simulink model "Thesis_VehicleModel_MPC_ECMS"  (R2018b)
settings: Solver=FixedStepAuto  StartTime=0.0  StopTime=10  FixedStep=0.01  RelTol=1e-5
PostLoadFcn:
  | , if any(exist('dsrtsu_mdlpostloadfcn', 'file') == [2, 3, 6]), try dsrtsu_mdlpostloadfcn('Execute', bdroot); catch fprintf('Error in PostLoadFcn (dsrtsu_mdlpostloadfcn) for model "%s":\n %s\n', bdroot, lasterr); end, end,
InitFcn:
  | clc;clear all;
model workspace (MAT data in the model file):
  MDL : struct (value not decoded)
values from neighbouring files (symbols this model uses):
  MDL =     [MDL.mat]
libraries: simulink x14, rtican x9, autolibshared x1, mpclib x1
(part 2 of 5)

== system Thesis_VehicleModel_MPC_ECMS/Genset Powertrain Dynamics2/Generator ==
  MechPwrIn(W) : Inport
  GensetCmd : Inport  Port=2
  Power Setpoint : Inport  Port=3
  Constant1 : Constant  Value=0
  Constant2 : Constant  Value=0
  Current Servo System : TransferFcn  Denominator=[0.2 1]
  Load Torque Servo System : TransferFcn  Denominator=[0.2 1]
  Product : Product
  Saturation : Saturate  UpperLimit=70  LowerLimit=0
  Saturation Dynamic : simulink/Discontinuities/Saturation Dynamic  OutMin=[]  OutMax=[]  OutDataTypeStr=Inherit: Same as second input  OutDataType=fixdt(1, 16)  OutScaling=2^-10  DoSatur=off
  Saturation Dynamic1 : simulink/Discontinuities/Saturation Dynamic  OutMin=[]  OutMax=[]  OutDataTypeStr=Inherit: Same as second input  OutDataType=fixdt(1, 16)  OutScaling=2^-10  DoSatur=off
  Saturation1 : Saturate  UpperLimit=inf  LowerLimit=0
  Subsystem : Subsystem
  Subtract : Sum  Inputs=+-
  Terminator : Terminator
  Thermal Contraint : Subsystem
  "Voltage, Current and Load Torque Mapping" : MATLAB Function  TreatAsAtomicUnit=on
  GenPwrOut (W) : Outport
  "Torque_Load " : Outport  Port=2
  MaxMechPwr : Outport  Port=3
  wires:
  GensetCmd/1 -> Subsystem/2("Genset Cmd ")
  Constant1/1 -> Saturation Dynamic/3
  Saturation Dynamic1/1 -> GenPwrOut (W)/1  "GenPwrOut (W)"
  Saturation Dynamic/1 -> Subtract/1, Subsystem/1(Mech_Pwr), Thermal Contraint/1(MechPwrIn)
  Thermal Contraint/1(MaxMechPwr) -> MaxMechPwr/1, Saturation Dynamic/1
  MechPwrIn(W)/1 -> Saturation Dynamic/2
  Subsystem/1(Pwr_Loss) -> Subtract/2  "Gen Pwr Loss"
  "Voltage, Current and Load Torque Mapping"/3(LoadTorque) -> Saturation/1  "T_load*"
  Load Torque Servo System/1 -> "Torque_Load "/1  "T_load"
  "Voltage, Current and Load Torque Mapping"/2(Current) -> Current Servo System/1  "Current*"
  Power Setpoint/1 -> "Voltage, Current and Load Torque Mapping"/1(P)  "Power_cmd"
  Saturation/1 -> Load Torque Servo System/1
  Constant2/1 -> Saturation Dynamic1/3
  Product/1 -> Saturation Dynamic1/2
  "Voltage, Current and Load Torque Mapping"/1(Volt) -> Product/2
  Current Servo System/1 -> Terminator/1, Product/1  "Current"
  Subtract/1 -> Saturation1/1
  Saturation1/1 -> Saturation Dynamic1/1  "Gen Upper Bound"

== system Thesis_VehicleModel_MPC_ECMS/Genset Powertrain Dynamics2/Power//rpm Setpoints ==
  Power Command : Inport
  Genset Cmd : Inport  Port=2
  Chart : Stateflow chart  TreatAsAtomicUnit=on
  Clock : Clock
  MATLAB Function : MATLAB Function  TreatAsAtomicUnit=on
  Power Setpoint : Outport
  rpm Setpoint : Outport  Port=2
  wires:
  Power Command/1 -> MATLAB Function/1(Power_Cmd)
  Clock/1 -> Chart/2(t)
  MATLAB Function/1(PowerSetPoint) -> Chart/1(PowerSetPoint)
  MATLAB Function/2(rpmSetPoint) -> Chart/3(rpmSetPoint)
  Chart/2(PowerCmd) -> Power Setpoint/1
  Chart/1(rpmCmd) -> rpm Setpoint/1
  Genset Cmd/1 -> MATLAB Function/2(GensetCmd)

== system Thesis_VehicleModel_MPC_ECMS/Genset Powertrain Dynamics2/Rpm Controller ==
  Engine rpm : Inport
  rpm setpoint : Inport  Port=2
  Engine Power Set Point : Inport  Port=3
  Calculate Feedback Mapping : Product  Multiplication=Matrix(*)
  Calculate Fix Point : Subsystem
  Demux : Demux  Outputs=2
  Gain : Gain  Gain=30/pi
  Kalman Filter : Subsystem
  LQG Gain Mapping : MATLAB Function  TreatAsAtomicUnit=on
  Noise : RandomNumber  Variance=300  SampleTime=0.1
  Scope : Scope
  Scope1 : Scope
  Sum : Sum  Inputs=|-+
  Sum1 : Sum  Inputs=|++
  Sum2 : Sum  Inputs=|++
  TPS limit : Saturate  UpperLimit=0.98  LowerLimit=0
  Terminator : Terminator
  dSPACE CANBUS Protocol : Subsystem  Commented=on
  rpm regulation : Stateflow chart  Commented=on  TreatAsAtomicUnit=on
  rpm2rads1 : Gain  Gain=pi/30
  TPS Command : Outport
  wires:
  Sum2/1 -> LQG Gain Mapping/1(rpm), rpm2rads1/1, Kalman Filter/2("rpm ")  "Engine rpm with noise"
  Kalman Filter/1("x_hat ") -> Scope/1, Sum/2, Gain/1  "State Estimation x_hat"
  Sum/1 -> Calculate Feedback Mapping/2
  Sum1/1 -> Kalman Filter/3(u)
  rpm2rads1/1 -> Kalman Filter/1(y)
  TPS limit/1 -> Sum1/2, TPS Command/1
  LQG Gain Mapping/2(gain) -> Calculate Feedback Mapping/1
  Engine rpm/1 -> Sum2/1
  Noise/1 -> Sum2/2
  LQG Gain Mapping/1(comp) -> Sum1/1
  rpm setpoint/1 -> Calculate Fix Point/1(rpm set point)
  Calculate Fix Point/1(rpm_cmd) -> LQG Gain Mapping/2(rpm_cmd)
  Calculate Fix Point/2(fix point (2 states)) -> Sum/1
  Engine Power Set Point/1 -> LQG Gain Mapping/3(PowerSetPoint)
  Calculate Feedback Mapping/1 -> TPS limit/1
  Gain/1 -> Demux/1
  Demux/1 -> Scope1/1
  Demux/2 -> Terminator/1

== system Thesis_VehicleModel_MPC_ECMS/RTI Data/RTI Data Store ==
  RTI Data Store : Subsystem  mask(RTI_DATA_STORE){}
      mask help:
      | RTI Data Store Block. This block is used by RTI to store internal model dependent data. Deleting this block will result in data loss.
      |
      | NEVER DELETE, COPY, OR MODIFY THIS BLOCK!
      mask Help:
      | RTI Data Store Block. This block is used by RTI to store internal model dependent data. Deleting this block will result in data loss.
      | 
      | NEVER DELETE, COPY, OR MODIFY THIS BLOCK!
      mask Display: text(0.5, 0.5, ' ', 'HorizontalAlignment', 'center');

== system Thesis_VehicleModel_MPC_ECMS/Supervisory Control MPC Archive/Nonlinear_MPC ==
  SOC : Inport
  SOC_ref : Inport  Port=2
  Measured Disturbance : Inport  Port=3
  Nonlinear MPC Controller1 : mpclib/Nonlinear MPC Controller  SCDEnableBlockLinearizationSpecification=on  nlmpcobj=Pw_Trobj  UseObjectTs=on  md_enabled=on  param_enabled=off  cost_enabled=on  mvseq_enabled=off  stateseq_enabled=off  ovseq_enabled=off  slack_enabled=off  status_enabled=on  ov_min=off  ov_max=off  mv_min=off  mv_max=off  mvrate_min=off  mvrate_max=off  state_min=off  state_max=off  ov_weight=off  mv_weight=off  mvrate_weight=off  ecr_weight=off  mvtarget_enabled=off  nlp_initialize=off
      settings: SourceProductName=Model Predictive Control Toolbox
  Terminator : Terminator
  Terminator1 : Terminator
  Unit Delay1 : UnitDelay  SampleTime=-1
  Manipulated Variable : Outport
  wires:
  Nonlinear MPC Controller1/1 -> Manipulated Variable/1, Unit Delay1/1
  Unit Delay1/1 -> Nonlinear MPC Controller1/3
  SOC/1 -> Nonlinear MPC Controller1/1
  SOC_ref/1 -> Nonlinear MPC Controller1/2
  Measured Disturbance/1 -> Nonlinear MPC Controller1/4
  Nonlinear MPC Controller1/2 -> Terminator/1  "MPC Optimal Cost"
  Nonlinear MPC Controller1/3 -> Terminator1/1  "MPC Status"

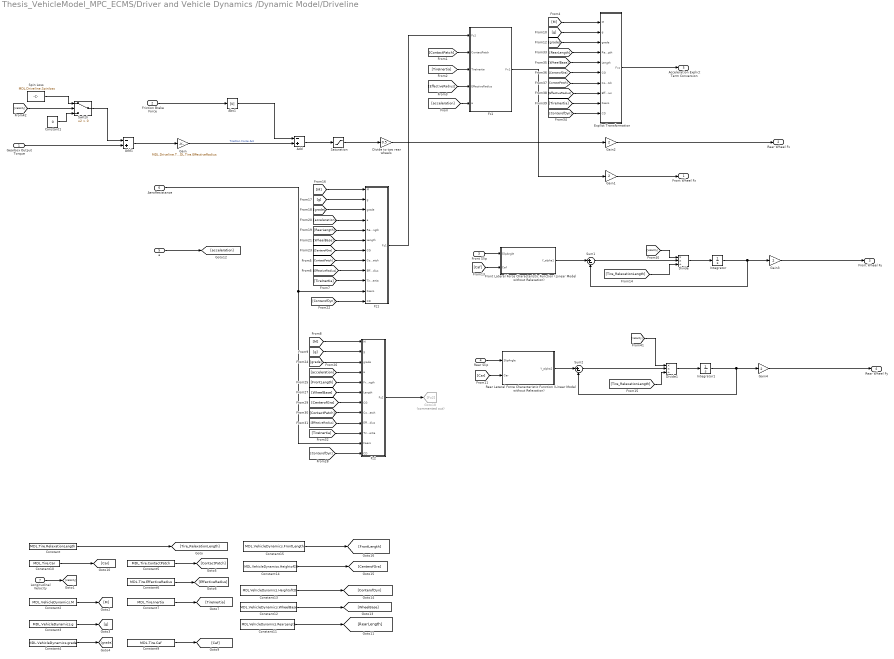
== system Thesis_VehicleModel_MPC_ECMS/Driver and Vehicle Dynamics /Dynamic Model/Driveline ==
  Gearbox Output Torque : Inport
  Friction Brake Force : Inport  Port=2
  Front Slip : Inport  Port=3
  Rear Slip : Inport  Port=4
  a : Inport  Port=5
  "AeroResistance " : Inport  Port=6
  Longitudinal Velocity : Inport  Port=7
  Abs1 : Abs
  Add : Sum  Inputs=-+
  Add1 : Sum  Inputs=-+
  Constant : Constant  Value=MDL.Tire.RelaxationLength
  Constant1 : Constant  Value=0
  Constant10 : Constant  Value=MDL.Tire.Car
  Constant11 : Constant  Value=MDL.VehicleDynamics.RearLength
  Constant12 : Constant  Value=MDL.VehicleDynamics.WheelBase
  Constant13 : Constant  Value=MDL.VehicleDynamics.HeightofCD
  Constant14 : Constant  Value=MDL.VehicleDynamics.HeightofCG
  Constant15 : Constant  Value=MDL.VehicleDynamics.FrontLength
  Constant2 : Constant  Value=MDL.VehicleDynamics.M
  Constant3 : Constant  Value=MDL.VehicleDynamics.g
  Constant4 : Constant  Value=MDL.VehicleDynamics.grade
  Constant5 : Constant  Value=MDL.Tire.ContactPatch
  Constant6 : Constant  Value=MDL.Tire.EffectiveRadius
  Constant7 : Constant  Value=MDL.Tire.Inertia
  Constant9 : Constant  Value=MDL.Tire.Caf
  Divide : Product  Inputs=**/
  Divide to two rear wheels : Gain  Gain=0.5
  Divide1 : Product  Inputs=**/
  Explict Transformation : MATLAB Function  TreatAsAtomicUnit=on
  Front Lateral Force Characteristic Function (Linear Model without Relexation) : MATLAB Function  TreatAsAtomicUnit=on
  Fx1 : MATLAB Function  TreatAsAtomicUnit=on
  Fz1 : MATLAB Function  TreatAsAtomicUnit=on
  Fz2 : MATLAB Function  TreatAsAtomicUnit=on
  Gain : Gain  Gain=MDL.Driveline.TFRatio/MDL.Tire.EffectiveRadius
  Gain{1..4} (4 alike) : Gain  Gain=2
  Goto18 : Goto  Commented=on  GotoTag=Fz2
  Integrator : Integrator
  Integrator1 : Integrator
  Rear Lateral Force Characteristic Function (Linear Model without Relexation) : MATLAB Function  TreatAsAtomicUnit=on
  Saturation : Saturate  UpperLimit=MDL.Driveline.MaxTrac  LowerLimit=-MDL.Driveline.MaxTrac
  Spin Loss : Constant  Value=MDL.Driveline.Spinloss
  Sum1 : Sum  Inputs=|+-
  Sum2 : Sum  Inputs=|+-
  Switch : Switch  Criteria=u2 > Threshold
  "Front Wheel Fx " : Outport
  Rear Wheel Fx : Outport  Port=2
  Front Wheel Fy : Outport  Port=3
  Rear Wheel Fy : Outport  Port=4
  Acceleration Explict Term Conversion : Outport  Port=5
  wires:
  Gearbox Output Torque/1 -> Add1/2
  Divide to two rear wheels/1 -> Gain2/1
  Front Slip/1 -> Front Lateral Force Characteristic Function (Linear Model without Relexation)/1(SlipAngle)
  Rear Slip/1 -> Rear Lateral Force Characteristic Function (Linear Model without Relexation)/1(SlipAngle)
  Gain1/1 -> "Front Wheel Fx "/1
  Gain2/1 -> Rear Wheel Fx/1
  Constant2/1 -> [M]
  Constant3/1 -> [g]
  Constant4/1 -> [grade]
  Constant5/1 -> [ContactPatch]
  Constant6/1 -> [EffectiveRadius]
  Constant7/1 -> [TireInertia]
  [ContactPatch] -> Fz1/8(ContactPatch)
  [EffectiveRadius] -> Fz1/9(EffectiveRadius)
  [TireInertia] -> Fz1/10(TireInertia)
  Constant9/1 -> [Caf]
  [Car] -> Rear Lateral Force Characteristic Function (Linear Model without Relexation)/2(Car)
  [Caf] -> Front Lateral Force Characteristic Function (Linear Model without Relexation)/2(Caf)
  Constant10/1 -> [Car]
  [M] -> Fz1/1(M)
  [g] -> Fz1/2(g)
  [grade] -> Fz1/3(grade)
  Constant11/1 -> [RearLength]
  [RearLength] -> Fz1/5(RearLength)
  [acceleration] -> Fz1/4(a)
  Constant12/1 -> [WheelBase]
  [WheelBase] -> Fz1/6(Length)
  Constant13/1 -> [ConterofDyn]
  [ConterofDyn] -> Fz1/12(CD)
  Constant14/1 -> [CenterofGra]
  [CenterofGra] -> Fz1/7(CG)
  [M] -> Fz2/1(M)
  [grade] -> Fz2/3(grade)
  [CenterofGra] -> Fz2/7(CG)
  [FrontLength] -> Fz2/5(FrontLength)
  [g] -> Fz2/2(g)
  [WheelBase] -> Fz2/6(Length)
  [EffectiveRadius] -> Fz2/9(EffectiveRadius)
  [ConterofDyn] -> Fz2/12(CD)
  [ContactPatch] -> Fz2/8(ContactPatch)
  [TireInertia] -> Fz2/10(TireInertia)
  [acceleration] -> Fz2/4(a)
  Constant15/1 -> [FrontLength]
  [ContactPatch] -> Fx1/2(ContactPatch)
  [TireInertia] -> Fx1/3(TireInertia)
  [EffectiveRadius] -> Fx1/4(EffectiveRadius)
  Fx1/1(Fx1) -> Gain1/1
  a/1 -> [acceleration]
  "AeroResistance "/1 -> Fz1/11(Faero), Fz2/11(Faero)
  Fz1/1(Fz1) -> Fx1/1(Fz1)
  [acceleration] -> Fx1/5(a)
  [M] -> Explict Transformation/1(M)
  [g] -> Explict Transformation/2(g)
  [grade] -> Explict Transformation/3(grade)
  [RearLength] -> Explict Transformation/4(RearLength)
  [WheelBase] -> Explict Transformation/5(Length)
  [CenterofGra] -> Explict Transformation/6(CG)
  [ContactPatch] -> Explict Transformation/7(ContactPatch)
  [EffectiveRadius] -> Explict Transformation/8(EffectiveRadius)
  [TireInertia] -> Explict Transformation/9(Faero)
  [ConterofDyn] -> Explict Transformation/10(CD)
  Explict Transformation/1(Fxs) -> Acceleration Explict Term Conversion/1
  Fz2/1(Fz2) -> Goto18/1
  Gain/1 -> Add/2  "Traction Force Acc"
  Integrator/1 -> Sum1/2, Gain3/1
  Front Lateral Force Characteristic Function (Linear Model without Relexation)/1(Y_alpha1) -> Sum1/1
  Constant/1 -> [Tire_RelexationLength]
  Sum1/1 -> Divide/2
  Divide/1 -> Integrator/1
  Gain3/1 -> Front Wheel Fy/1
  Integrator1/1 -> Sum2/2, Gain4/1
  Sum2/1 -> Divide1/2
  Divide1/1 -> Integrator1/1
  Rear Lateral Force Characteristic Function (Linear Model without Relexation)/1(Y_alpha2) -> Sum2/1
  Gain4/1 -> Rear Wheel Fy/1
  [Tire_RelexationLength] -> Divide1/3
  [Tire_RelexationLength] -> Divide/3
  [Velocity] -> Divide/1
  Longitudinal Velocity/1 -> [Velocity]
  [Velocity] -> Divide1/1
  Friction Brake Force/1 -> Abs1/1
  Abs1/1 -> Add/1
  Add/1 -> Saturation/1
  Saturation/1 -> Divide to two rear wheels/1
  Add1/1 -> Gain/1
  [Velocity] -> Switch/2
  Constant1/1 -> Switch/3
  Switch/1 -> Add1/1
  Spin Loss/1 -> Switch/1

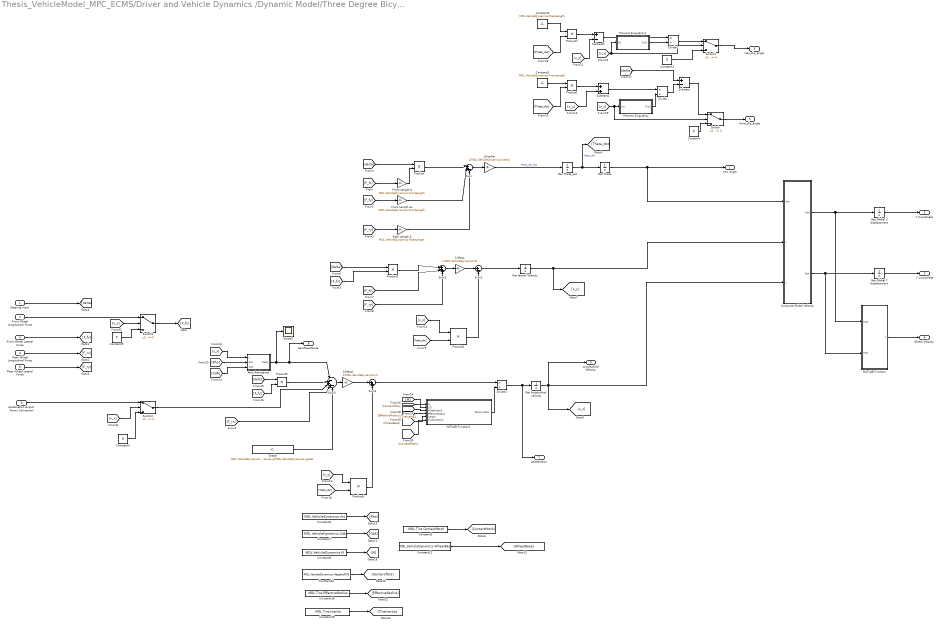
== system Thesis_VehicleModel_MPC_ECMS/Driver and Vehicle Dynamics /Dynamic Model/Three Degree Bicycle Model ==
  Steering Input : Inport
  Front Wheel Longitudinal Force : Inport  Port=2
  Rear Wheel Longitudinal Force : Inport  Port=3
  Front Wheel Lateral Force : Inport  Port=4
  Rear Wheel Lateral Force : Inport  Port=5
  Acceleration Explict Terms Conversion : Inport  Port=6
  1/Inertia : Gain  Gain=1/MDL.VehicleDynamics.Inertia
  1/Mass : Gain  Gain=1/MDL.VehicleDynamics.M
  1/Mass1 : Gain  Gain=1/MDL.VehicleDynamics.M
  Aero Resistance : MATLAB Function  TreatAsAtomicUnit=on
  Compute Global Velocity : MATLAB Function  TreatAsAtomicUnit=on
  Constant{,1,4,9} (4 alike) : Constant  Value=0
  Constant12 : Constant  Value=MDL.VehicleDynamics.WheelBase
  Constant14 : Constant  Value=MDL.VehicleDynamics.HeightofCG
  Constant18 : Constant  Value=MDL.Tire.EffectiveRadius
  Constant19 : Constant  Value=MDL.Tire.Inertia
  Constant2 : Constant  Value=MDL.VehicleDynamics.RearLength
  Constant3 : Constant  Value=MDL.VehicleDynamics.FrontLength
  Constant5 : Constant  Value=MDL.Tire.ContactPatch
  Constant6 : Constant  Value=MDL.VehicleDynamics.rho
  Constant7 : Constant  Value=MDL.VehicleDynamics.CdA
  Constant8 : Constant  Value=MDL.VehicleDynamics.M
  Divide : Product  Inputs=*/
  Divide1 : Product  Inputs=*/
  Divide2 : Product  Inputs=*/
  Front Length a : Gain  Gain=MDL.VehicleDynamics.FrontLength
  Front Length a1 : Gain  Gain=MDL.VehicleDynamics.FrontLength
  Get Global X displacement : Integrator
  Get Global Y displacement : Integrator
  Get Theta : Integrator
  Get Theta_dot : Integrator
  Get lateral Velocity : Integrator
  Get longitudinal velocity : Integrator
  Grade : Constant  Value=MDL.VehicleDynamics.M*MDL.VehicleDynamics.g*MDL.VehicleDynamics.grade
  MATLAB Function : MATLAB Function  TreatAsAtomicUnit=on
  MATLAB Function1 : MATLAB Function  TreatAsAtomicUnit=on
  Prevent Singularity : Subsystem
  Prevent Singularity1 : Subsystem
  Product{,1..3,5..7} (7 alike) : Product
  Rear Length b : Gain  Gain=MDL.VehicleDynamics.RearLength
  Scope2 : Scope
  Subtract : Sum  Inputs=+-
  Subtract1 : Sum  Inputs=+-
  Subtract2 : Sum
  Sum : Sum  Inputs=|++-
  Sum1 : Sum  Inputs=|+++
  Sum2 : Sum  Inputs=|+-
  Sum3 : Sum  Inputs=|--++-
  Sum4 : Sum  Inputs=|++
  Switch{,1..3} (4 alike) : Switch  Criteria=u2 ~= 0
  Yaw Angle : Outport
  Y Coordinate : Outport  Port=2
  X Coordinate : Outport  Port=3
  Global Velocity : Outport  Port=4
  front_slip_angle : Outport  Port=5
  rear_slip_angle : Outport  Port=6
  Acceleration : Outport  Port=7
  "AeroResistance " : Outport  Port=8
  "Longitudinal Velocity " : Outport  Port=9
  wires:
  [F_ry] -> Sum1/3
  1/Inertia/1 -> Get Theta_dot/1  "Theta_dot_dot"
  Get Theta_dot/1 -> [Theta_dot], Get Theta/1  "Theta_dot"
  Sum3/1 -> 1/Mass1/1
  [Theta_dot] -> Product3/2
  [delta] -> Product2/1
  Product2/1 -> Sum1/1
  [Theta_dot] -> Product6/2
  [v_y] -> Product6/1
  Product6/1 -> Sum4/2
  [delta] -> Product5/1
  Sum/1 -> 1/Inertia/1
  [F_fy] -> Sum1/2
  Get lateral Velocity/1 -> Compute Global Velocity/2(v), [v_y]
  Rear Wheel Longitudinal Force/1 -> [F_rx]
  [F_fy] -> Product5/2
  Steering Input/1 -> [delta]
  Front Wheel Lateral Force/1 -> [F_fy]
  [F_fx] -> Front Length a/1
  [F_fy] -> Front Length a1/1
  Front Wheel Longitudinal Force/1 -> Switch3/1
  Rear Wheel Lateral Force/1 -> [F_ry]
  Sum1/1 -> 1/Mass/1
  Get longitudinal velocity/1 -> "Longitudinal Velocity "/1, Compute Global Velocity/3(u), [v_x]
  [F_ry] -> Rear Length b/1
  Product3/1 -> Sum2/2
  [v_x] -> Product3/1
  Rear Length b/1 -> Sum/3
  1/Mass/1 -> Sum2/1
  Product/1 -> Sum/1
  Front Length a1/1 -> Sum/2
  Front Length a/1 -> Product/2
  Sum2/1 -> Get lateral Velocity/1
  Constant3/1 -> Product1/1
  [Theta_dot] -> Product1/2
  Product1/1 -> Subtract2/1
  [v_y] -> Subtract2/2
  Subtract2/1 -> Divide/1
  [v_x] -> Switch/2, Prevent Singularity/1(In1)
  [delta] -> Subtract/1
  Divide/1 -> Subtract/2
  Constant2/1 -> Product7/1
  [Theta_dot] -> Product7/2
  Product7/1 -> Subtract1/1
  [v_y] -> Subtract1/2
  Subtract1/1 -> Divide1/1
  Switch/1 -> front_slip_angle/1
  Subtract/1 -> Switch/1
  Constant/1 -> Switch/3
  Switch1/1 -> rear_slip_angle/1
  Divide1/1 -> Switch1/1
  Constant1/1 -> Switch1/3
  [delta] -> Product/1
  Get Global Y displacement/1 -> Y Coordinate/1
  Get Theta/1 -> Yaw Angle/1, Compute Global Velocity/1(Yaw)
  Compute Global Velocity/2(Ydot) -> MATLAB Function/2(Ydot), Get Global Y displacement/1
  Compute Global Velocity/1(Xdot) -> MATLAB Function/1(Xdot), Get Global X displacement/1
  Get Global X displacement/1 -> X Coordinate/1
  MATLAB Function/1(V) -> Global Velocity/1
  [v_x] -> Aero Resistance/1(u)
  [F_rx] -> Sum3/4
  Product5/1 -> Sum3/2
  Aero Resistance/1(Faero) -> Scope2/1, "AeroResistance "/1, Sum3/1
  [CdA] -> Aero Resistance/3(CdA)
  [Rho] -> Aero Resistance/2(Rho)
  1/Mass1/1 -> Sum4/1
  Constant14/1 -> [CenterofGra]
  Constant7/1 -> [CdA]
  Constant18/1 -> [EffectiveRadius]
  Constant19/1 -> [TireInertia]
  Constant8/1 -> [M]
  Constant6/1 -> [Rho]
  Divide2/1 -> Get longitudinal velocity/1, Acceleration/1
  [M] -> MATLAB Function1/1(M)
  [CenterofGra] -> MATLAB Function1/2(CG)
  [TireInertia] -> MATLAB Function1/3(WheelInertia)
  [EffectiveRadius] -> MATLAB Function1/4(EffectiveRadius)
  [WheelBase] -> MATLAB Function1/5(Length)
  Constant12/1 -> [WheelBase]
  Sum4/1 -> Divide2/1
  MATLAB Function1/1(Denominator) -> Divide2/2
  Constant5/1 -> [ContactPatch]
  [ContactPatch] -> MATLAB Function1/6(ContactPatch)
  [v_x] -> Switch1/2, Prevent Singularity1/1(In1)
  Prevent Singularity1/1(Out1) -> Divide1/2
  [v_x] -> Switch2/2
  Constant4/1 -> Switch2/3
  Switch2/1 -> Sum3/3
  Acceleration Explict Terms Conversion/1 -> Switch2/1
  [F_fx] -> Product2/2
  [v_x] -> Switch3/2
  Constant9/1 -> Switch3/3
  Switch3/1 -> [F_fx]
  Prevent Singularity/1(Out1) -> Divide/2
  Grade/1 -> Sum3/5

== system Thesis_VehicleModel_MPC_ECMS/Driver and Vehicle Dynamics /EMRAX Motor Model /Brake System ==
  "BPP " : Inport
  V (m/s) : Inport  Port=2
  Bus Creator : BusCreator  Inputs=2
  Constant : Constant  Value=0
  Gain : Gain  Gain=MDL.BrakeSys.MaxBrakeForce
  Gain1 : Gain  Gain=1-MDL.BrakeSys.RegenFraction
  Gain2 : Gain  Gain=MDL.BrakeSys.RegenFraction
  Gain3 : Gain  Gain=10
  Gain4 : Gain  Gain=MDL.Tire.EffectiveRadius/MDL.VehicleDynamics.g
  Product : Product  RndMeth=Zero
  Saturation : Saturate  UpperLimit=1  LowerLimit=0  ZeroCross=off
  Scope : Scope
  Switch : Switch  Criteria=u2 > Threshold
  Switch1 : Switch  Criteria=u2 > Threshold
  BrakeCmd : Outport
  wires:
  Bus Creator/1 -> BrakeCmd/1
  "BPP "/1 -> Gain/1
  Gain/1 -> Gain1/1, Gain2/1  "Desired Brake Force"
  Gain2/1 -> Gain4/1  "Regen Brake Force"
  Gain1/1 -> Switch1/1  "Friction Brake Force"
  Product/1 -> Switch/1  "Regen Brake Torque"
  V (m/s)/1 -> Gain3/1, Switch/2, Switch1/2
  Saturation/1 -> Product/2
  Gain3/1 -> Saturation/1
  Gain4/1 -> Product/1
  Switch/1 -> Bus Creator/2  "Regen Brake Torque"
  Constant/1 -> Switch/3, Switch1/3
  Switch1/1 -> Scope/1, Bus Creator/1  "Friction Brake Force"

== system Thesis_VehicleModel_MPC_ECMS/Driver and Vehicle Dynamics /EMRAX Motor Model /EMRAX 228 Motor ==
  Regen Brake Torque Cmd : Inport
  APP : Inport  Port=2
  Motor Speed (rad/s) : Inport  Port=3
  1-D Lookup Table : Lookup_n-D  NumberOfTableDimensions=1  BreakpointsForDimension1=[0,2000,3000,4000,5000,5500,6500]  Table=[240,240,234,228,216,100,0]  InternalRulePriority=Speed  OutMin=[0]  OutMax=[250]  RndMeth=Simplest  InputSameDT=on
  2-D Lookup Table : Lookup_n-D  LookupTableObject=Map  BreakpointsForDimension1=MDL.MotorModel.EffMapTorque  BreakpointsForDimension2=MDL.MotorModel.EffMapRPM  Table=MDL.MotorModel.EffMapData  InternalRulePriority=Speed  RndMeth=Simplest  InputSameDT=on
  Abs : Abs
  Add : Sum
  Divide : Product  Inputs=/*
  Gain1 : Gain  Gain=-1
  MATLAB Function : MATLAB Function  TreatAsAtomicUnit=on
  Product2 : Product
  Product3 : Product
  Saturation : Saturate  UpperLimit=1  LowerLimit=0.10
  Saturation Dynamic : simulink/Discontinuities/Saturation Dynamic  OutMin=[]  OutMax=[]  OutDataTypeStr=Inherit: Same as second input  OutDataType=fixdt(1, 16)  OutScaling=2^-10  DoSatur=off
  "Spin Loss " : MATLAB Function  TreatAsAtomicUnit=on
  Sum : Sum  Inputs=|++
  rad2rpm : Gain  Gain=30/pi
  Motor Torque : Outport
  Power_Consumption : Outport  Port=2
  wires:
  APP/1 -> Product2/1
  Saturation Dynamic/1 -> Sum/1, Abs/1, Product3/1
  Product3/1 -> MATLAB Function/2(P_mot), Divide/2  "Power Output"
  Divide/1 -> Power_Consumption/1
  Product2/1 -> Add/2
  Add/1 -> Saturation Dynamic/2
  [Toc_LocMax] -> Saturation Dynamic/1
  [Toc_LocMax] -> Gain1/1
  Gain1/1 -> Saturation Dynamic/3
  2-D Lookup Table/1 -> Saturation/1  "Motor Efficiency"
  Motor Speed (rad/s)/1 -> Product3/2, rad2rpm/1
  1-D Lookup Table/1 -> Product2/2, [Toc_LocMax]
  Regen Brake Torque Cmd/1 -> Add/1
  Abs/1 -> 2-D Lookup Table/1
  rad2rpm/1 -> 1-D Lookup Table/1, 2-D Lookup Table/2, "Spin Loss "/1(omega)  "Motor rpm"
  "Spin Loss "/1(T_sl) -> Sum/2
  Sum/1 -> Motor Torque/1
  MATLAB Function/1(Efficiency) -> Divide/1
  Saturation/1 -> MATLAB Function/1(Eff)

== system Thesis_VehicleModel_MPC_ECMS/Genset Powertrain Dynamics/Battery/DP_Battery_Model ==
  Current : Inport
  Open Circuit Voltage : Inport  Port=2
  Cpa : Constant  Value=5630*6
  Cpc : Constant  Value=54277*6
  Divide : Product  Inputs=*//
  Divide1 : Product  Inputs=*/
  Divide2 : Product  Inputs=*//
  Divide3 : Product  Inputs=*/
  Gain : Gain  Gain=-1
  Gain1 : Gain  Gain=-1
  Integrator : Integrator
  Integrator1 : Integrator
  Product : Product
  "Ro " : Constant  Value=0.06
  Rpa : Constant  Value=0.00064
  Rpc : Constant  Value=0.00839
  Sum : Sum  Inputs=|++
  Sum1 : Sum  Inputs=|++
  Sum2 : Sum  Inputs=+---
  Terminal Voltage : Outport
  wires:
  Rpa/1 -> Divide/3
  Cpa/1 -> Divide1/2, Divide/2
  Sum/1 -> Integrator/1
  Product/1 -> Sum2/2
  Divide/1 -> Gain/1
  "Ro "/1 -> Product/1
  Sum2/1 -> Terminal Voltage/1
  Open Circuit Voltage/1 -> Sum2/1
  Divide1/1 -> Sum/1
  Gain/1 -> Sum/2
  Sum1/1 -> Integrator1/1
  Divide2/1 -> Gain1/1
  Divide3/1 -> Sum1/1
  Integrator/1 -> Sum2/3, Divide/1  "Upa"
  Integrator1/1 -> Sum2/4, Divide2/1  "Upc"
  Current/1 -> Product/2, Divide1/1, Divide3/1
  Cpc/1 -> Divide3/2, Divide2/2
  Rpc/1 -> Divide2/3
  Gain1/1 -> Sum1/2

== system Thesis_VehicleModel_MPC_ECMS/Genset Powertrain Dynamics/Engine/Engine_Dynamics  ==
  "Torque_load " : Inport
  TPS Command : Inport  Port=2
  1/Shaft_Inertia : Gain  Gain=1/0.73
  Closed throttle torque : MATLAB Function  TreatAsAtomicUnit=on
  Engine rpm-torque map : Lookup_n-D  NumberOfTableDimensions=1  BreakpointsForDimension1=[0,800,1000,1500,2000,2500,3000,3500,4000,4500,5000,6500]  Table=[100,100,105,115,125,132,136,140,142,139,135,0]  InternalRulePriority=Speed  OutMin=[0]  OutMax=[150]  RndMeth=Simplest  InputSameDT=on
  Integrator : Integrator  LimitOutput=on  LowerSaturationLimit=0
  Product : Product
  Saturation2 : Saturate  UpperLimit=1  LowerLimit=0
  Sum : Sum  Inputs=+-+
  Throttle_subsystem : TransferFcn  Denominator=[0.2 1]
  rads2rpm : Gain  Gain=30/pi
  Engine torque : Outport
  Eng_rpm : Outport  Port=2
  wires:
  Throttle_subsystem/1 -> Saturation2/1
  Engine rpm-torque map/1 -> Product/2
  [Eng_rpm] -> Engine rpm-torque map/1
  TPS Command/1 -> Throttle_subsystem/1
  Product/1 -> Engine torque/1, Sum/1  "T_eng"
  Saturation2/1 -> Product/1  "TPS"
  Integrator/1 -> Closed throttle torque/1(w), rads2rpm/1
  Sum/1 -> 1/Shaft_Inertia/1
  1/Shaft_Inertia/1 -> Integrator/1
  Closed throttle torque/1(T) -> Sum/3
  rads2rpm/1 -> [Eng_rpm], Eng_rpm/1
  "Torque_load "/1 -> Sum/2  "T_load"

== system Thesis_VehicleModel_MPC_ECMS/Genset Powertrain Dynamics/Engine/Fuel_Consumption ==
  note: Fuel Consumption
  Genset_Cmd : Inport
  Engine Torque : Inport  Port=2
  EngPwrOut(W) : Inport  Port=3
  Engine rpm : Inport  Port=4
  Add3 : Sum
  Add4 : Sum
  Detect Increase : simulink/Logic and Bit Operations/Detect Increase  vinit=0.0  OutDataTypeStr=uint8
  Divide : Product  Inputs=*/
  Engine Efficiency Map : Lookup_n-D  BreakpointsForDimension1=MDL.EngineModel.EffMapTorque  BreakpointsForDimension2=MDL.EngineModel.EffMapRPM  Table=3600/46.4./MDL.EngineModel.EffMapData  InternalRulePriority=Speed  RndMeth=Simplest  InputSameDT=on
  Gain3 : Gain  Gain=MDL.EngineModel.EngStartEnergy
  Gain4 : Gain  Gain=1/MDL.EngineModel.LHV
  Integrator2 : Integrator
  Memory : Memory
  Saturation : Saturate  UpperLimit=1  LowerLimit=0
  Fuel Consumption(g) : Outport
  wires:
  Memory/1 -> Add3/1
  Add3/1 -> Memory/1, Gain3/1
  Detect Increase/1 -> Add3/2
  Gain4/1 -> Fuel Consumption(g)/1  "Fuel Consumption"
  [GensetCmd] -> Detect Increase/1
  Add4/1 -> Gain4/1  "Energy(J)"
  Integrator2/1 -> Add4/2
  Gain3/1 -> Add4/1
  Divide/1 -> Integrator2/1  "Pwr_Eng"
  Genset_Cmd/1 -> [GensetCmd]
  Engine Torque/1 -> Engine Efficiency Map/1
  Engine rpm/1 -> Engine Efficiency Map/2
  Engine Efficiency Map/1 -> Saturation/1
  EngPwrOut(W)/1 -> Divide/1
  Saturation/1 -> Divide/2

== system Thesis_VehicleModel_MPC_ECMS/Genset Powertrain Dynamics/Generator/Subsystem ==
  Mech_Pwr : Inport
  "Genset Cmd " : Inport  Port=2
  Add1 : Sum  Inputs=+++
  Constant2 : Constant  Value=0
  Constant3 : Constant  Value=MDL.GeneratorModel.C0
  Gain1 : Gain  Gain=MDL.GeneratorModel.C1
  Gain2 : Gain  Gain=MDL.GeneratorModel.C2
  Math Function : Math  Operator=square  SaturateOnIntegerOverflow=on
  Switch : Switch
  Pwr_Loss : Outport
  wires:
  Mech_Pwr/1 -> Math Function/1, Gain1/1
  Constant3/1 -> Switch/1
  Add1/1 -> Pwr_Loss/1
  Gain1/1 -> Add1/2
  Gain2/1 -> Add1/3
  [GensetCmd] -> Switch/2
  Switch/1 -> Add1/1
  Constant2/1 -> Switch/3
  Math Function/1 -> Gain2/1
  "Genset Cmd "/1 -> [GensetCmd]

== system Thesis_VehicleModel_MPC_ECMS/Genset Powertrain Dynamics/Generator/Thermal Contraint ==
  MechPwrIn : Inport
  Add : Sum  Inputs=+-
  Compare To Constant : simulink/Logic and Bit Operations/Compare To Constant  relop=<=  const=3.0  OutDataTypeStr=boolean
  Constant1 : Constant  Value=MDL.GeneratorModel.ContMechPwr
  Constant2 : Constant  Value=MDL.GeneratorModel.ContMechPwr
  Constant3 : Constant  Value=MDL.GeneratorModel.PeakMechPwr
  Gain : Gain  Gain=1/(MDL.GeneratorModel.PeakMechPwr-MDL.GeneratorModel.ContMechPwr)
  Gain1 : Gain  Gain=1/60
  Integrator : Integrator  LimitOutput=on  UpperSaturationLimit=1  LowerSaturationLimit=0
  Switch1 : Switch  Criteria=u2 ~= 0
  MaxMechPwr : Outport
  wires:
  MechPwrIn/1 -> Add/1
  Constant2/1 -> Add/2
  Add/1 -> Gain/1
  Gain/1 -> Gain1/1
  Gain1/1 -> Integrator/1
  Integrator/1 -> Compare To Constant/1
  Compare To Constant/1 -> Switch1/2
  Constant1/1 -> Switch1/1
  Constant3/1 -> Switch1/3
  Switch1/1 -> MaxMechPwr/1

== system Thesis_VehicleModel_MPC_ECMS/Genset Powertrain Dynamics/Rpm Controller/Calculate Fix Point ==
  rpm set point : Inport
  Constant1 : Constant  Value=0
  Mux : Mux  Inputs=2
  Saturation : Saturate  UpperLimit=6000  LowerLimit=0
  rpm2rads : Gain  Gain=pi/30
  rpm_cmd : Outport
  fix point (2 states) : Outport  Port=2
  wires:
  Constant1/1 -> Mux/2
  Mux/1 -> rpm2rads/1
  rpm set point/1 -> Saturation/1
  Saturation/1 -> Mux/1, rpm_cmd/1
  rpm2rads/1 -> fix point (2 states)/1

== system Thesis_VehicleModel_MPC_ECMS/Genset Powertrain Dynamics/Rpm Controller/Kalman Filter ==
  y : Inport
  "rpm " : Inport  Port=2
  u : Inport  Port=3
  Bu : MATLAB Function  TreatAsAtomicUnit=on
  Engine rpm-torque map : Lookup_n-D  NumberOfTableDimensions=1  BreakpointsForDimension1=[800,1000,1500,2000,2500,3000,3500,4000,4500,5000,6500]  Table=[100,105,115,125,132,136,140,142,139,135,0]  InternalRulePriority=Speed  RndMeth=Simplest  InputSameDT=on
  Gain : Gain  Gain=MDL.ThrottleController.KFL  Multiplication=Matrix(K*u)
  Gain2 : Gain  Gain=MDL.ThrottleController.KFA  Multiplication=Matrix(K*u)
  Gain4 : Gain  Gain=MDL.ThrottleController.KFC  Multiplication=Matrix(K*u)
  Integrator : Integrator
  Sum1 : Sum  Inputs=|+++
  Sum2 : Sum  Inputs=|+-
  "x_hat " : Outport
  wires:
  Sum1/1 -> Integrator/1
  Gain4/1 -> Sum2/2
  Gain/1 -> Sum1/2
  Integrator/1 -> Gain4/1, Gain2/1, "x_hat "/1
  Bu/1(y) -> Sum1/1
  Gain2/1 -> Sum1/3
  Sum2/1 -> Gain/1
  y/1 -> Sum2/1
  u/1 -> Bu/1(u)
  "rpm "/1 -> Engine rpm-torque map/1
  Engine rpm-torque map/1 -> Bu/2(Tmax)
